simulink model "fuzzy_controller_5_trimf_optimal"  (R2016a)
settings: Solver=ode45  StartTime=0.0  StopTime=10.0  RelTol=1e-3
values from neighbouring files (symbols this model uses):
  FORCE_Range_1 = -150    [fuzzy_controller_3_trimf_params.m]    (also in fuzzy_controller_5_gauss_params.m; fuzzy_controller_5_gbell_params.m; fuzzy_controller_5_trimf_optimal_params.m; fuzzy_controller_5_trimf_params.m)
  FORCE_Range_2 = 150    [fuzzy_controller_3_trimf_params.m]    (also in fuzzy_controller_5_gauss_params.m; fuzzy_controller_5_gbell_params.m; fuzzy_controller_5_trimf_optimal_params.m; fuzzy_controller_5_trimf_params.m)
undefined symbols (not defined in the file): fi_1_a, fi_1_b, fi_1_c, fi_1_d, fi_2_a, fi_2_b, fi_2_c, fi_3_a, fi_3_b, fi_3_c, fi_4_a, fi_4_b, fi_4_c, fi_5_a, fi_5_b, fi_5_c, fi_5_d, FORCE_1_a, FORCE_1_b, FORCE_1_c, FORCE_2_a, FORCE_2_b, FORCE_2_c, FORCE_3_a, FORCE_3_b, FORCE_3_c, FORCE_4_a, FORCE_4_b, FORCE_4_c, FORCE_5_a, FORCE_5_b, FORCE_5_c, omega_1_a, omega_1_b, omega_1_c, omega_1_d, omega_2_a, omega_2_b, omega_2_c, omega_3_a, omega_3_b, omega_3_c, omega_4_a, omega_4_b, omega_4_c, omega_5_a, omega_5_b, omega_5_c, omega_5_d
libraries: fuzblock x40, fuzwiz x2
(part 2 of 2)

== system fuzzy_controller_5_trimf_optimal/Fuzzy Logic Controller/fi/tri mf4 ==
  x : Inport
  If : If  IfExpression=(u1<a) | (u1>c)  ElseIfExpressions=u1==b, u1 < b  ZeroCross=off
  If Action Subsystem : fuzblock/Membership  Functions/Triangular MF/If Action Subsystem
  If Action Subsystem1 : fuzblock/Membership  Functions/Triangular MF/If Action Subsystem1
  If Action Subsystem2 : fuzblock/Membership  Functions/Triangular MF/If Action Subsystem2
  If Action Subsystem3 : fuzblock/Membership  Functions/Triangular MF/If Action Subsystem3
  Merge : Merge  Inputs=4
  MF : Outport
  wires:
  If Action Subsystem3/1 -> Merge/3
  If/3 -> If Action Subsystem3/Action
  If Action Subsystem2/1 -> Merge/4
  If/4 -> If Action Subsystem2/Action
  If Action Subsystem1/1 -> Merge/2
  If/2 -> If Action Subsystem1/Action
  If Action Subsystem/1 -> Merge/1
  Merge/1 -> MF/1
  If/1 -> If Action Subsystem/Action
  x/1 -> If Action Subsystem3/1, If Action Subsystem2/1, If/1

== system fuzzy_controller_5_trimf_optimal/Fuzzy Logic Controller/omega/trap mf1 ==
  x : Inport
  If Action Subsystem : fuzblock/Membership  Functions/Triangular MF/If Action Subsystem
  If Action Subsystem1 : fuzblock/Membership  Functions/Triangular MF/If Action Subsystem1
  If Action Subsystem2 : fuzblock/Membership  Functions/Trapezoidal MF/If Action Subsystem1
  If Action Subsystem8 : fuzblock/Membership  Functions/Trapezoidal MF/If Action Subsystem3
  If2 : If  IfExpression=(u1 < a) | (u1>d)  ElseIfExpressions=(u1 >= b) & (u1 <= c), u1 < b  ZeroCross=off
  Merge : Merge  Inputs=4
  MF : Outport
  wires:
  If Action Subsystem2/1 -> Merge/3
  If2/3 -> If Action Subsystem2/Action
  If Action Subsystem8/1 -> Merge/4
  If2/4 -> If Action Subsystem8/Action
  If Action Subsystem1/1 -> Merge/2
  If2/2 -> If Action Subsystem1/Action
  If Action Subsystem/1 -> Merge/1
  Merge/1 -> MF/1
  If2/1 -> If Action Subsystem/Action
  x/1 -> If Action Subsystem2/1, If Action Subsystem8/1, If2/1

== system fuzzy_controller_5_trimf_optimal/Fuzzy Logic Controller/omega/trap mf5 ==
  x : Inport
  If Action Subsystem : fuzblock/Membership  Functions/Triangular MF/If Action Subsystem
  If Action Subsystem1 : fuzblock/Membership  Functions/Triangular MF/If Action Subsystem1
  If Action Subsystem2 : fuzblock/Membership  Functions/Trapezoidal MF/If Action Subsystem1
  If Action Subsystem8 : fuzblock/Membership  Functions/Trapezoidal MF/If Action Subsystem3
  If2 : If  IfExpression=(u1 < a) | (u1>d)  ElseIfExpressions=(u1 >= b) & (u1 <= c), u1 < b  ZeroCross=off
  Merge : Merge  Inputs=4
  MF : Outport
  wires:
  If Action Subsystem2/1 -> Merge/3
  If2/3 -> If Action Subsystem2/Action
  If Action Subsystem8/1 -> Merge/4
  If2/4 -> If Action Subsystem8/Action
  If Action Subsystem1/1 -> Merge/2
  If2/2 -> If Action Subsystem1/Action
  If Action Subsystem/1 -> Merge/1
  Merge/1 -> MF/1
  If2/1 -> If Action Subsystem/Action
  x/1 -> If Action Subsystem2/1, If Action Subsystem8/1, If2/1

== system fuzzy_controller_5_trimf_optimal/Fuzzy Logic Controller/omega/tri mf2 ==
  x : Inport
  If : If  IfExpression=(u1<a) | (u1>c)  ElseIfExpressions=u1==b, u1 < b  ZeroCross=off
  If Action Subsystem : fuzblock/Membership  Functions/Triangular MF/If Action Subsystem
  If Action Subsystem1 : fuzblock/Membership  Functions/Triangular MF/If Action Subsystem1
  If Action Subsystem2 : fuzblock/Membership  Functions/Triangular MF/If Action Subsystem2
  If Action Subsystem3 : fuzblock/Membership  Functions/Triangular MF/If Action Subsystem3
  Merge : Merge  Inputs=4
  MF : Outport
  wires:
  If Action Subsystem3/1 -> Merge/3
  If/3 -> If Action Subsystem3/Action
  If Action Subsystem2/1 -> Merge/4
  If/4 -> If Action Subsystem2/Action
  If Action Subsystem1/1 -> Merge/2
  If/2 -> If Action Subsystem1/Action
  If Action Subsystem/1 -> Merge/1
  Merge/1 -> MF/1
  If/1 -> If Action Subsystem/Action
  x/1 -> If Action Subsystem3/1, If Action Subsystem2/1, If/1

== system fuzzy_controller_5_trimf_optimal/Fuzzy Logic Controller/omega/tri mf3 ==
  x : Inport
  If : If  IfExpression=(u1<a) | (u1>c)  ElseIfExpressions=u1==b, u1 < b  ZeroCross=off
  If Action Subsystem : fuzblock/Membership  Functions/Triangular MF/If Action Subsystem
  If Action Subsystem1 : fuzblock/Membership  Functions/Triangular MF/If Action Subsystem1
  If Action Subsystem2 : fuzblock/Membership  Functions/Triangular MF/If Action Subsystem2
  If Action Subsystem3 : fuzblock/Membership  Functions/Triangular MF/If Action Subsystem3
  Merge : Merge  Inputs=4
  MF : Outport
  wires:
  If Action Subsystem3/1 -> Merge/3
  If/3 -> If Action Subsystem3/Action
  If Action Subsystem2/1 -> Merge/4
  If/4 -> If Action Subsystem2/Action
  If Action Subsystem1/1 -> Merge/2
  If/2 -> If Action Subsystem1/Action
  If Action Subsystem/1 -> Merge/1
  Merge/1 -> MF/1
  If/1 -> If Action Subsystem/Action
  x/1 -> If Action Subsystem3/1, If Action Subsystem2/1, If/1

== system fuzzy_controller_5_trimf_optimal/Fuzzy Logic Controller/omega/tri mf4 ==
  x : Inport
  If : If  IfExpression=(u1<a) | (u1>c)  ElseIfExpressions=u1==b, u1 < b  ZeroCross=off
  If Action Subsystem : fuzblock/Membership  Functions/Triangular MF/If Action Subsystem
  If Action Subsystem1 : fuzblock/Membership  Functions/Triangular MF/If Action Subsystem1
  If Action Subsystem2 : fuzblock/Membership  Functions/Triangular MF/If Action Subsystem2
  If Action Subsystem3 : fuzblock/Membership  Functions/Triangular MF/If Action Subsystem3
  Merge : Merge  Inputs=4
  MF : Outport
  wires:
  If Action Subsystem3/1 -> Merge/3
  If/3 -> If Action Subsystem3/Action
  If Action Subsystem2/1 -> Merge/4
  If/4 -> If Action Subsystem2/Action
  If Action Subsystem1/1 -> Merge/2
  If/2 -> If Action Subsystem1/Action
  If Action Subsystem/1 -> Merge/1
  Merge/1 -> MF/1
  If/1 -> If Action Subsystem/Action
  x/1 -> If Action Subsystem3/1, If Action Subsystem2/1, If/1
